simulink model "dft_polyphase_channelizer_32_by_8"  (R2018b)
settings: Solver=FixedStepDiscrete  StartTime=0.0  StopTime=t(end)  RelTol=1e-3  EnableMultiTasking=on
InitFcn:
  | M = 32; % Number of channels in the filter bank.
  | N = 8;  % Number of taps in each FIR filter.
  | n_out = 4000; % Number of output samples
  | datatypeselector = 'hdl'; % 'double' 'single' 'hdl' 'dsp'
  | fidatatype = 'Fixed'; % 'Fixed' 'ScaledDouble'
  | [T,B,U,b,u,t,fs] = generate_inputs(M,N,n_out,datatypeselector,fidatatype);
values from neighbouring files (symbols this model uses):
  B = cast(B,'like',T.fir_filter.coeff)    [generate_inputs.m]
  fs = n    [generate_inputs.m]
  T = dft_polyphase_filter_types(datatypeselector,fidatatype,prototypevalue,max(abs(b)))    [generate_inputs.m]
(part 2 of 2)

== matlab function dft_polyphase_channelizer_32_by_8/Uniform Discrete Fourier Transform Polyphase Filter Bank/ CORDIC Complex to Magnitude Angle8 ==
  data: Z input; magnitudeZ output; angleZ output
function [magnitudeZ, angleZ] = cordic_magnitude_angle(Z)
    [magnitudeZ, angleZ] = cordic_cart2pol(Z);
end

== matlab function dft_polyphase_channelizer_32_by_8/Uniform Discrete Fourier Transform Polyphase Filter Bank/ CORDIC Complex to Magnitude Angle9 ==
  data: Z input; magnitudeZ output; angleZ output
function [magnitudeZ, angleZ] = cordic_magnitude_angle(Z)
    [magnitudeZ, angleZ] = cordic_cart2pol(Z);
end

== matlab function dft_polyphase_channelizer_32_by_8/Uniform Discrete Fourier Transform Polyphase Filter Bank/FFT/IFFT MATLAB Implementation ==
  data: X input; Y output; T parameter
function Y = inverse_fft_block(X,T)
    dim = 1;
    Y = inverse_fft(X, T, dim);
end

== matlab function dft_polyphase_channelizer_32_by_8/Uniform Discrete Fourier Transform Polyphase Filter Bank/FIR Filter 1 ==
  data: u input; x output; b parameter; T parameter
function x = fir_filter(u, b, T)
    persistent p z
    if isempty(p)
        p = zeros(1,'like',T.p);
        z = zeros(size(b),'like',T.z);
    end
    [x,z,p] = fir_filter_circular_buffer(b,u,z,p,T);
end

== matlab function dft_polyphase_channelizer_32_by_8/Uniform Discrete Fourier Transform Polyphase Filter Bank/FIR Filter 10 ==
  data: u input; x output; b parameter; T parameter
function x = fir_filter(u, b, T)
    persistent p z
    if isempty(p)
        p = zeros(1,'like',T.p);
        z = zeros(size(b),'like',T.z);
    end
    [x,z,p] = fir_filter_circular_buffer(b,u,z,p,T);
end

== matlab function dft_polyphase_channelizer_32_by_8/Uniform Discrete Fourier Transform Polyphase Filter Bank/FIR Filter 11 ==
  data: u input; x output; b parameter; T parameter
function x = fir_filter(u, b, T)
    persistent p z
    if isempty(p)
        p = zeros(1,'like',T.p);
        z = zeros(size(b),'like',T.z);
    end
    [x,z,p] = fir_filter_circular_buffer(b,u,z,p,T);
end

== matlab function dft_polyphase_channelizer_32_by_8/Uniform Discrete Fourier Transform Polyphase Filter Bank/FIR Filter 12 ==
  data: u input; x output; b parameter; T parameter
function x = fir_filter(u, b, T)
    persistent p z
    if isempty(p)
        p = zeros(1,'like',T.p);
        z = zeros(size(b),'like',T.z);
    end
    [x,z,p] = fir_filter_circular_buffer(b,u,z,p,T);
end

== matlab function dft_polyphase_channelizer_32_by_8/Uniform Discrete Fourier Transform Polyphase Filter Bank/FIR Filter 13 ==
  data: u input; x output; b parameter; T parameter
function x = fir_filter(u, b, T)
    persistent p z
    if isempty(p)
        p = zeros(1,'like',T.p);
        z = zeros(size(b),'like',T.z);
    end
    [x,z,p] = fir_filter_circular_buffer(b,u,z,p,T);
end

== matlab function dft_polyphase_channelizer_32_by_8/Uniform Discrete Fourier Transform Polyphase Filter Bank/FIR Filter 14 ==
  data: u input; x output; b parameter; T parameter
function x = fir_filter(u, b, T)
    persistent p z
    if isempty(p)
        p = zeros(1,'like',T.p);
        z = zeros(size(b),'like',T.z);
    end
    [x,z,p] = fir_filter_circular_buffer(b,u,z,p,T);
end

== matlab function dft_polyphase_channelizer_32_by_8/Uniform Discrete Fourier Transform Polyphase Filter Bank/FIR Filter 15 ==
  data: u input; x output; b parameter; T parameter
function x = fir_filter(u, b, T)
    persistent p z
    if isempty(p)
        p = zeros(1,'like',T.p);
        z = zeros(size(b),'like',T.z);
    end
    [x,z,p] = fir_filter_circular_buffer(b,u,z,p,T);
end

== matlab function dft_polyphase_channelizer_32_by_8/Uniform Discrete Fourier Transform Polyphase Filter Bank/FIR Filter 16 ==
  data: u input; x output; b parameter; T parameter
function x = fir_filter(u, b, T)
    persistent p z
    if isempty(p)
        p = zeros(1,'like',T.p);
        z = zeros(size(b),'like',T.z);
    end
    [x,z,p] = fir_filter_circular_buffer(b,u,z,p,T);
end

== matlab function dft_polyphase_channelizer_32_by_8/Uniform Discrete Fourier Transform Polyphase Filter Bank/FIR Filter 17 ==
  data: u input; x output; b parameter; T parameter
function x = fir_filter(u, b, T)
    persistent p z
    if isempty(p)
        p = zeros(1,'like',T.p);
        z = zeros(size(b),'like',T.z);
    end
    [x,z,p] = fir_filter_circular_buffer(b,u,z,p,T);
end

== matlab function dft_polyphase_channelizer_32_by_8/Uniform Discrete Fourier Transform Polyphase Filter Bank/FIR Filter 18 ==
  data: u input; x output; b parameter; T parameter
function x = fir_filter(u, b, T)
    persistent p z
    if isempty(p)
        p = zeros(1,'like',T.p);
        z = zeros(size(b),'like',T.z);
    end
    [x,z,p] = fir_filter_circular_buffer(b,u,z,p,T);
end

== matlab function dft_polyphase_channelizer_32_by_8/Uniform Discrete Fourier Transform Polyphase Filter Bank/FIR Filter 19 ==
  data: u input; x output; b parameter; T parameter
function x = fir_filter(u, b, T)
    persistent p z
    if isempty(p)
        p = zeros(1,'like',T.p);
        z = zeros(size(b),'like',T.z);
    end
    [x,z,p] = fir_filter_circular_buffer(b,u,z,p,T);
end

== matlab function dft_polyphase_channelizer_32_by_8/Uniform Discrete Fourier Transform Polyphase Filter Bank/FIR Filter 2 ==
  data: u input; x output; b parameter; T parameter
function x = fir_filter(u, b, T)
    persistent p z
    if isempty(p)
        p = zeros(1,'like',T.p);
        z = zeros(size(b),'like',T.z);
    end
    [x,z,p] = fir_filter_circular_buffer(b,u,z,p,T);
end

== matlab function dft_polyphase_channelizer_32_by_8/Uniform Discrete Fourier Transform Polyphase Filter Bank/FIR Filter 20 ==
  data: u input; x output; b parameter; T parameter
function x = fir_filter(u, b, T)
    persistent p z
    if isempty(p)
        p = zeros(1,'like',T.p);
        z = zeros(size(b),'like',T.z);
    end
    [x,z,p] = fir_filter_circular_buffer(b,u,z,p,T);
end

== matlab function dft_polyphase_channelizer_32_by_8/Uniform Discrete Fourier Transform Polyphase Filter Bank/FIR Filter 21 ==
  data: u input; x output; b parameter; T parameter
function x = fir_filter(u, b, T)
    persistent p z
    if isempty(p)
        p = zeros(1,'like',T.p);
        z = zeros(size(b),'like',T.z);
    end
    [x,z,p] = fir_filter_circular_buffer(b,u,z,p,T);
end

== matlab function dft_polyphase_channelizer_32_by_8/Uniform Discrete Fourier Transform Polyphase Filter Bank/FIR Filter 22 ==
  data: u input; x output; b parameter; T parameter
function x = fir_filter(u, b, T)
    persistent p z
    if isempty(p)
        p = zeros(1,'like',T.p);
        z = zeros(size(b),'like',T.z);
    end
    [x,z,p] = fir_filter_circular_buffer(b,u,z,p,T);
end

== matlab function dft_polyphase_channelizer_32_by_8/Uniform Discrete Fourier Transform Polyphase Filter Bank/FIR Filter 23 ==
  data: u input; x output; b parameter; T parameter
function x = fir_filter(u, b, T)
    persistent p z
    if isempty(p)
        p = zeros(1,'like',T.p);
        z = zeros(size(b),'like',T.z);
    end
    [x,z,p] = fir_filter_circular_buffer(b,u,z,p,T);
end

== matlab function dft_polyphase_channelizer_32_by_8/Uniform Discrete Fourier Transform Polyphase Filter Bank/FIR Filter 24 ==
  data: u input; x output; b parameter; T parameter
function x = fir_filter(u, b, T)
    persistent p z
    if isempty(p)
        p = zeros(1,'like',T.p);
        z = zeros(size(b),'like',T.z);
    end
    [x,z,p] = fir_filter_circular_buffer(b,u,z,p,T);
end

== matlab function dft_polyphase_channelizer_32_by_8/Uniform Discrete Fourier Transform Polyphase Filter Bank/FIR Filter 25 ==
  data: u input; x output; b parameter; T parameter
function x = fir_filter(u, b, T)
    persistent p z
    if isempty(p)
        p = zeros(1,'like',T.p);
        z = zeros(size(b),'like',T.z);
    end
    [x,z,p] = fir_filter_circular_buffer(b,u,z,p,T);
end

== matlab function dft_polyphase_channelizer_32_by_8/Uniform Discrete Fourier Transform Polyphase Filter Bank/FIR Filter 26 ==
  data: u input; x output; b parameter; T parameter
function x = fir_filter(u, b, T)
    persistent p z
    if isempty(p)
        p = zeros(1,'like',T.p);
        z = zeros(size(b),'like',T.z);
    end
    [x,z,p] = fir_filter_circular_buffer(b,u,z,p,T);
end

== matlab function dft_polyphase_channelizer_32_by_8/Uniform Discrete Fourier Transform Polyphase Filter Bank/FIR Filter 27 ==
  data: u input; x output; b parameter; T parameter
function x = fir_filter(u, b, T)
    persistent p z
    if isempty(p)
        p = zeros(1,'like',T.p);
        z = zeros(size(b),'like',T.z);
    end
    [x,z,p] = fir_filter_circular_buffer(b,u,z,p,T);
end

== matlab function dft_polyphase_channelizer_32_by_8/Uniform Discrete Fourier Transform Polyphase Filter Bank/FIR Filter 28 ==
  data: u input; x output; b parameter; T parameter
function x = fir_filter(u, b, T)
    persistent p z
    if isempty(p)
        p = zeros(1,'like',T.p);
        z = zeros(size(b),'like',T.z);
    end
    [x,z,p] = fir_filter_circular_buffer(b,u,z,p,T);
end

== matlab function dft_polyphase_channelizer_32_by_8/Uniform Discrete Fourier Transform Polyphase Filter Bank/FIR Filter 29 ==
  data: u input; x output; b parameter; T parameter
function x = fir_filter(u, b, T)
    persistent p z
    if isempty(p)
        p = zeros(1,'like',T.p);
        z = zeros(size(b),'like',T.z);
    end
    [x,z,p] = fir_filter_circular_buffer(b,u,z,p,T);
end

== matlab function dft_polyphase_channelizer_32_by_8/Uniform Discrete Fourier Transform Polyphase Filter Bank/FIR Filter 3 ==
  data: u input; x output; b parameter; T parameter
function x = fir_filter(u, b, T)
    persistent p z
    if isempty(p)
        p = zeros(1,'like',T.p);
        z = zeros(size(b),'like',T.z);
    end
    [x,z,p] = fir_filter_circular_buffer(b,u,z,p,T);
end

== matlab function dft_polyphase_channelizer_32_by_8/Uniform Discrete Fourier Transform Polyphase Filter Bank/FIR Filter 30 ==
  data: u input; x output; b parameter; T parameter
function x = fir_filter(u, b, T)
    persistent p z
    if isempty(p)
        p = zeros(1,'like',T.p);
        z = zeros(size(b),'like',T.z);
    end
    [x,z,p] = fir_filter_circular_buffer(b,u,z,p,T);
end

== matlab function dft_polyphase_channelizer_32_by_8/Uniform Discrete Fourier Transform Polyphase Filter Bank/FIR Filter 31 ==
  data: u input; x output; b parameter; T parameter
function x = fir_filter(u, b, T)
    persistent p z
    if isempty(p)
        p = zeros(1,'like',T.p);
        z = zeros(size(b),'like',T.z);
    end
    [x,z,p] = fir_filter_circular_buffer(b,u,z,p,T);
end

== matlab function dft_polyphase_channelizer_32_by_8/Uniform Discrete Fourier Transform Polyphase Filter Bank/FIR Filter 32 ==
  data: u input; x output; b parameter; T parameter
function x = fir_filter(u, b, T)
    persistent p z
    if isempty(p)
        p = zeros(1,'like',T.p);
        z = zeros(size(b),'like',T.z);
    end
    [x,z,p] = fir_filter_circular_buffer(b,u,z,p,T);
end

== matlab function dft_polyphase_channelizer_32_by_8/Uniform Discrete Fourier Transform Polyphase Filter Bank/FIR Filter 4 ==
  data: u input; x output; b parameter; T parameter
function x = fir_filter(u, b, T)
    persistent p z
    if isempty(p)
        p = zeros(1,'like',T.p);
        z = zeros(size(b),'like',T.z);
    end
    [x,z,p] = fir_filter_circular_buffer(b,u,z,p,T);
end

== matlab function dft_polyphase_channelizer_32_by_8/Uniform Discrete Fourier Transform Polyphase Filter Bank/FIR Filter 5 ==
  data: u input; x output; b parameter; T parameter
function x = fir_filter(u, b, T)
    persistent p z
    if isempty(p)
        p = zeros(1,'like',T.p);
        z = zeros(size(b),'like',T.z);
    end
    [x,z,p] = fir_filter_circular_buffer(b,u,z,p,T);
end

== matlab function dft_polyphase_channelizer_32_by_8/Uniform Discrete Fourier Transform Polyphase Filter Bank/FIR Filter 6 ==
  data: u input; x output; b parameter; T parameter
function x = fir_filter(u, b, T)
    persistent p z
    if isempty(p)
        p = zeros(1,'like',T.p);
        z = zeros(size(b),'like',T.z);
    end
    [x,z,p] = fir_filter_circular_buffer(b,u,z,p,T);
end

== matlab function dft_polyphase_channelizer_32_by_8/Uniform Discrete Fourier Transform Polyphase Filter Bank/FIR Filter 7 ==
  data: u input; x output; b parameter; T parameter
function x = fir_filter(u, b, T)
    persistent p z
    if isempty(p)
        p = zeros(1,'like',T.p);
        z = zeros(size(b),'like',T.z);
    end
    [x,z,p] = fir_filter_circular_buffer(b,u,z,p,T);
end

== matlab function dft_polyphase_channelizer_32_by_8/Uniform Discrete Fourier Transform Polyphase Filter Bank/FIR Filter 8 ==
  data: u input; x output; b parameter; T parameter
function x = fir_filter(u, b, T)
    persistent p z
    if isempty(p)
        p = zeros(1,'like',T.p);
        z = zeros(size(b),'like',T.z);
    end
    [x,z,p] = fir_filter_circular_buffer(b,u,z,p,T);
end

== matlab function dft_polyphase_channelizer_32_by_8/Uniform Discrete Fourier Transform Polyphase Filter Bank/FIR Filter 9 ==
  data: u input; x output; b parameter; T parameter
function x = fir_filter(u, b, T)
    persistent p z
    if isempty(p)
        p = zeros(1,'like',T.p);
        z = zeros(size(b),'like',T.z);
    end
    [x,z,p] = fir_filter_circular_buffer(b,u,z,p,T);
end
